simulink model "Assignment_2"  (R2025b)
settings: Solver=VariableStepAuto  StartTime=0.0  StopTime=1000  RelTol=1e-3
undefined symbols (not defined in the file): dspblkCoreblockFVToolHelper, gcbh
libraries: simulink x6, dspinverses x2, androidaudiovideolib x1, androiduilib x1, dspstat3 x1
settings Model: Creator=vishr  LastModifiedBy=vishr

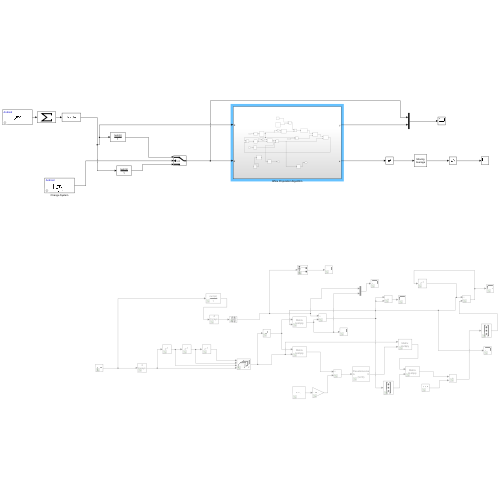
[thumbnail: Simulink's stored preview of the top-level diagram]
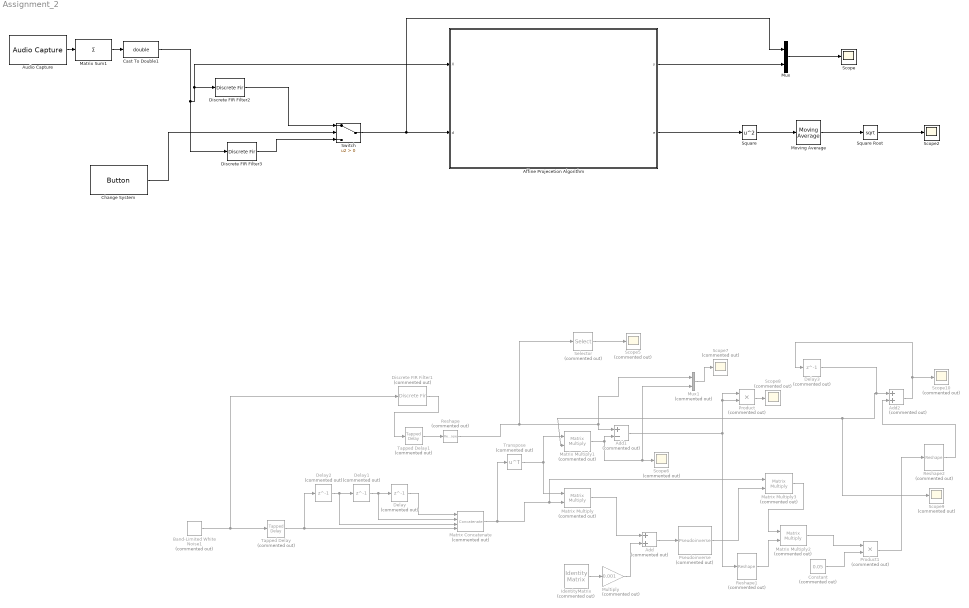
== system Assignment_2 ==
  Add : Sum  Commented=on
  Add1 : Sum  Commented=on  Inputs=+-  InputSameDT=on
  Add2 : Sum  Commented=on
  Affine Projecetion Algorithm : Subsystem
  Audio Capture : androidaudiovideolib/Audio Capture  SampleFreq=44100  FrameSize=4410  SampleTime=0.1  SimulateUsing=Code generation  DeviceStr=0  QueueDuration=0  BlockPlatform=Android  AudioSamplingFreq=44100
  Band-Limited White Noise1 : simulink/Sources/Band-Limited White Noise  Commented=on  Cov=[0.1]  Ts=0.1  seed=[23341]
  Cast To Double1 : DataTypeConversion  OutDataTypeStr=double  SaturateOnIntegerOverflow=off  RndMeth=Floor
  Change System : androiduilib/Button  ButtonState=Not pressed  ButtonId=Assignment_2/Change_System  State=off  SampleTime=0.1  BlockPlatform=Android
  Constant : Constant  Commented=on  Value=0.05
  Delay{,1..3} (4 alike) : Delay  Commented=on  DelayLength=1  InputProcessing=Columns as channels (frame based)
  Discrete FIR Filter1 : DiscreteFir  Commented=on  LoadFcn=dspblkCoreblockFVToolHelper(gcbh,'load');  Coefficients=[0.2 0.4 -0.7 0.1]
      settings: CopyFcn=dspblkCoreblockFVToolHelper(gcbh,'copy');  DeleteFcn=dspblkCoreblockFVToolHelper(gcbh,'close');  ModelCloseFcn=dspblkCoreblockFVToolHelper(gcbh,'close');  PreSaveFcn=dspblkCoreblockFVToolHelper(gcbh,'presave');  PostSaveFcn=dspblkCoreblockFVToolHelper(gcbh,'postsave');  CloseFcn=dspblkCoreblockFVToolHelper(gcbh,'close');
  Discrete FIR Filter2 : DiscreteFir  LoadFcn=dspblkCoreblockFVToolHelper(gcbh,'load');  Coefficients=[0.1 0.2 -0.3 0.8 0.4 -0.1]
      settings: CopyFcn=dspblkCoreblockFVToolHelper(gcbh,'copy');  DeleteFcn=dspblkCoreblockFVToolHelper(gcbh,'close');  ModelCloseFcn=dspblkCoreblockFVToolHelper(gcbh,'close');  PreSaveFcn=dspblkCoreblockFVToolHelper(gcbh,'presave');  PostSaveFcn=dspblkCoreblockFVToolHelper(gcbh,'postsave');  CloseFcn=dspblkCoreblockFVToolHelper(gcbh,'close');
  Discrete FIR Filter3 : DiscreteFir  LoadFcn=dspblkCoreblockFVToolHelper(gcbh,'load');  Coefficients=[-0.1 0.3 0.9 0.5 0.8 -0.3]
      settings: CopyFcn=dspblkCoreblockFVToolHelper(gcbh,'copy');  DeleteFcn=dspblkCoreblockFVToolHelper(gcbh,'close');  ModelCloseFcn=dspblkCoreblockFVToolHelper(gcbh,'close');  PreSaveFcn=dspblkCoreblockFVToolHelper(gcbh,'presave');  PostSaveFcn=dspblkCoreblockFVToolHelper(gcbh,'postsave');  CloseFcn=dspblkCoreblockFVToolHelper(gcbh,'close');
  IdentityMatrix : IdentityMatrix  Commented=on  OutputDimensions=4
  Matrix Concatenate : Concatenate  Commented=on  NumInputs=4  Mode=Multidimensional array  ConcatenateDimension=2
  Matrix Sum1 : Sum  Inputs=+
  Matrix Multiply{,1..3} (4 alike) : Product  Commented=on  Multiplication=Matrix(*)
  Moving Average : dspstat3/Moving Average  Method=Sliding window  ForgettingFactorPort=off  SpecifyWindowLength=on  WindowLength=4  OverlapLength=3  AllowArbitraryInputLength=off  ForgettingFactor=0.9  SimulateUsing=Interpreted execution
  Multiply : Gain  Commented=on  Gain=0.001
  Mux : Mux  Inputs=2
  Mux1 : Mux  Commented=on  Inputs=2
  Product : Product  Commented=on
  Product1 : Product  Commented=on
  Pseudoinverse : dspinverses/Pseudoinverse  Commented=on  wanterr=off  SimulateUsing=Interpreted execution
  Reshape : Reshape  Commented=on  OutputDimensionality=Column vector (2-D)
  Reshape1 : Reshape  Commented=on  OutputDimensionality=Column vector (2-D)
  Reshape2 : Reshape  Commented=on  OutputDimensionality=Column vector (2-D)
  Scope : Scope
      settings: ActiveDisplayYMinimum=-89266.988167443342  ActiveDisplayYMaximum=136454.23417264404  DataLoggingVariableName=ScopeData2
  Scope{5..10} (6 alike) : Scope  Commented=on
      Scope10 settings: ActiveDisplayYMinimum=-1  ActiveDisplayYMaximum=1  DataLoggingVariableName=ScopeData10
      Scope5 settings: ActiveDisplayYMinimum=-2.8115847650322072  ActiveDisplayYMaximum=3.0353378563712785  DataLoggingVariableName=ScopeData5
      Scope6 settings: DataLoggingVariableName=ScopeData6
      Scope7 settings: ActiveDisplayYMinimum=-1  ActiveDisplayYMaximum=1  DataLoggingVariableName=ScopeData7
      Scope8 settings: DataLoggingVariableName=ScopeData8
      Scope9 settings: ActiveDisplayYMinimum=-1  ActiveDisplayYMaximum=1  DataLoggingVariableName=ScopeData9
  Scope2 : Scope
      settings: ActiveDisplayYMinimum=0  ActiveDisplayYMaximum=1.5
  Selector : Selector  Commented=on  InputPortWidth=4  IndexOptions=Index vector (dialog)  Indices=[1 3]  OutputSizes=1
  Square : Math  Operator=square
  Square Root : Sqrt
  Switch : Switch  Criteria=u2 > Threshold  SaturateOnIntegerOverflow=off  InputSameDT=off
  Tapped Delay : simulink/Discrete/Tapped Delay  Commented=on  vinit=0.0  samptime=-1  NumDelays=2  DelayOrder=Oldest  includeCurrent=off
  Tapped Delay1 : simulink/Discrete/Tapped Delay  Commented=on  vinit=0.0  samptime=-1  NumDelays=4  DelayOrder=Oldest  includeCurrent=off
  Transpose : Math  Commented=on  Operator=transpose
  wires:
  Affine Projecetion Algorithm/1(y) -> Mux/2
  Affine Projecetion Algorithm/2(e) -> Square/1
  Mux/1 -> Scope/1
  Square/1 -> Moving Average/1
  Moving Average/1 -> Square Root/1
  Delay/1 -> Matrix Concatenate/1
  Delay2/1 -> Matrix Concatenate/3, Delay1/1
  Delay1/1 -> Matrix Concatenate/2, Delay/1
  Tapped Delay/1 -> Delay2/1, Matrix Concatenate/4
  IdentityMatrix/1 -> Multiply/1
  Multiply/1 -> Add/2
  Matrix Multiply/1 -> Add/1
  Matrix Concatenate/1 -> Transpose/1, Matrix Multiply3/1, Matrix Multiply/2
  Band-Limited White Noise1/1 -> Discrete FIR Filter1/1, Tapped Delay/1
  Transpose/1 -> Matrix Multiply1/1, Matrix Multiply/1
  Matrix Multiply1/1 -> Mux1/2, Scope6/1, Add1/2
  Add/1 -> Pseudoinverse/1
  Pseudoinverse/1 -> Matrix Multiply3/2
  Matrix Multiply3/1 -> Matrix Multiply2/1
  Add1/1 -> Reshape1/1, Product/1, Product/2
  Mux1/1 -> Scope7/1
  Product/1 -> Scope8/1
  Delay3/1 -> Scope9/1, Matrix Multiply1/2, Add2/1
  Add2/1 -> Delay3/1, Scope10/1
  Matrix Multiply2/1 -> Product1/1
  Constant/1 -> Product1/2
  Product1/1 -> Reshape2/1
  Reshape/1 -> Selector/1, Mux1/1, Add1/1
  Discrete FIR Filter1/1 -> Tapped Delay1/1
  Reshape2/1 -> Add2/2
  Reshape1/1 -> Matrix Multiply2/2
  Tapped Delay1/1 -> Reshape/1
  Selector/1 -> Scope5/1
  Square Root/1 -> Scope2/1
  Cast To Double1/1 -> Discrete FIR Filter3/1, Affine Projecetion Algorithm/1(X), Discrete FIR Filter2/1
  Change System/1 -> Switch/2
  Matrix Sum1/1 -> Cast To Double1/1
  Audio Capture/1 -> Matrix Sum1/1
  Discrete FIR Filter3/1 -> Switch/3
  Discrete FIR Filter2/1 -> Switch/1
  Switch/1 -> Mux/1, Affine Projecetion Algorithm/2(d)

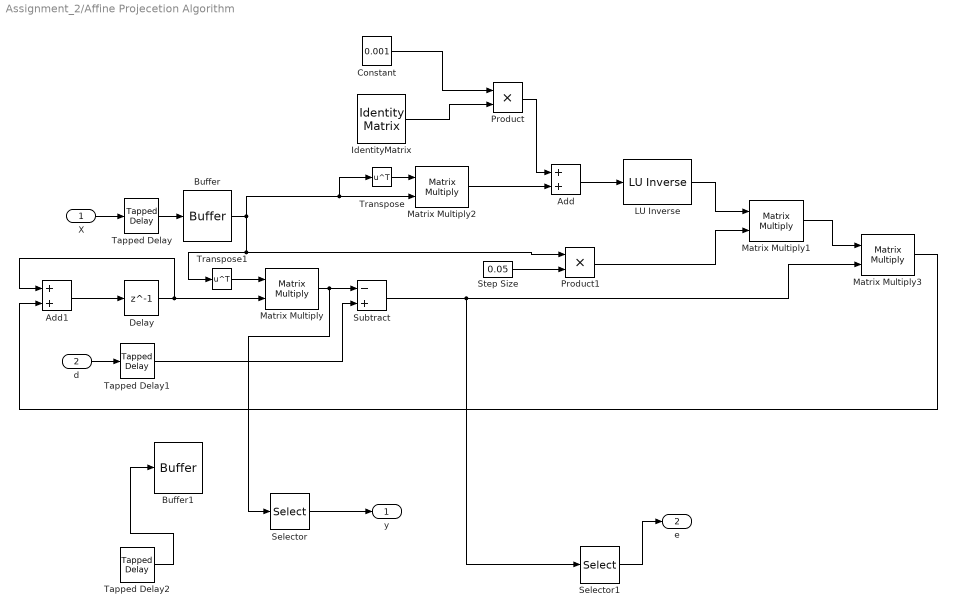
== system Assignment_2/Affine Projecetion Algorithm ==
  X : Inport
  d : Inport  Port=2
  " LU Inverse" : dspinverses/ LU Inverse
  Add : Sum
  Add1 : Sum
  Buffer : Buffer  N=6  OutputFrames=off
  Buffer1 : Buffer  N=6  OutputFrames=off
  Constant : Constant  Value=0.001
  Delay : Delay  DelayLength=1  InputProcessing=Columns as channels (frame based)
  IdentityMatrix : IdentityMatrix  OutputDimensions=6
  Matrix Multiply{,1..3} (4 alike) : Product  Multiplication=Matrix(*)
  Product : Product
  Product1 : Product
  Selector : Selector  InputPortWidth=6  IndexOptions=Index vector (dialog)  Indices=1  OutputSizes=1
  Selector1 : Selector  InputPortWidth=6  IndexOptions=Index vector (dialog)  Indices=1  OutputSizes=1
  Step Size : Constant  Value=0.05
  Subtract : Sum  Inputs=-+
  Tapped Delay : simulink/Discrete/Tapped Delay  vinit=0.0  samptime=-1  NumDelays=6  DelayOrder=Oldest  includeCurrent=off
  Tapped Delay1 : simulink/Discrete/Tapped Delay  vinit=0.0  samptime=-1  NumDelays=6  DelayOrder=Oldest  includeCurrent=off
  Tapped Delay2 : simulink/Discrete/Tapped Delay  vinit=0.0  samptime=-1  NumDelays=6  DelayOrder=Oldest  includeCurrent=off
  Transpose : Math  Operator=transpose
  Transpose1 : Math  Operator=transpose
  y : Outport
  e : Outport  Port=2
  wires:
  Tapped Delay1/1 -> Subtract/2
  Product1/1 -> Matrix Multiply1/2
  Matrix Multiply1/1 -> Matrix Multiply3/1
  Matrix Multiply3/1 -> Add1/2
  Product/1 -> Add/1
  Matrix Multiply/1 -> Selector/1, Subtract/1
  Tapped Delay/1 -> Buffer/1
  " LU Inverse"/1 -> Matrix Multiply1/1
  Matrix Multiply2/1 -> Add/2
  Buffer/1 -> Product1/1, Transpose1/1, Matrix Multiply2/2, Transpose/1
  Step Size/1 -> Product1/2
  Add/1 -> " LU Inverse"/1
  Add1/1 -> Delay/1
  Delay/1 -> Add1/1, Matrix Multiply/2
  Constant/1 -> Product/1
  X/1 -> Tapped Delay/1
  Subtract/1 -> Selector1/1, Matrix Multiply3/2
  Transpose/1 -> Matrix Multiply2/1
  Transpose1/1 -> Matrix Multiply/1
  IdentityMatrix/1 -> Product/2
  Selector/1 -> y/1
  Selector1/1 -> e/1
  d/1 -> Tapped Delay1/1
  Tapped Delay2/1 -> Buffer1/1
